simulink model "lvpp2d"  (Simulink 8.4)
settings: Solver=ode45  SolverMode=SingleTasking  StartTime=0.0  StopTime=20  RelTol=1e-3  AbsTol=1e-6
settings Model: Creator=The MathWorks Inc.  LastModifiedBy=gcampa  ExtModeTrigMode=oneshot  ExtModeArmWhenConnect=off
settings DataIOCC: ExternalInput=[]  InitialState=[]  LimitDataPoints=off  SaveOutput=off  SaveTime=off
settings OptimizationCC: BlockReduction=off  BooleanDataType=off  ExpressionDepthLimit=128  InitFltsAndDblsToZero=on
settings DebuggingCC: SaveWithParameterizedLinksMsg=none  SignalResolutionControl=TryResolveAllWithWarning  SolverPrmCheckMsg=none  MultiTaskDSMMsg=warning  MultiTaskCondExecSysMsg=none  IntegerOverflowMsg=none  FcnCallInpInsideContextMsg=EnableAllAsError  FrameProcessingCompatibilityMsg=error  StateNameClashWarn=none
settings HardwareCC: TargetUnknown=on
settings GRTTargetCC: TargetFcnLib=ansi_tfl_tmw.mat
settings ConfigComp: CovMetricSettings=dw  CovHtmlReporting=on  CovSaveCumulativeToWorkspaceVar=on  CovSaveSingleToWorkspaceVar=on  CovModelRefEnable=Off  CovExternalEMLEnable=off  CovSFcnEnable=off

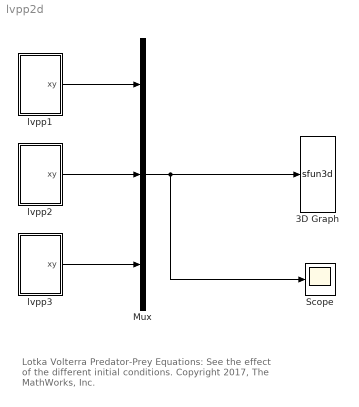
== system lvpp2d ==
  note: Lotka Volterra Predator-Prey Equations:
      | See the effect of the different initial conditions.
      | Copyright 2017, The MathWorks, Inc.
  3D Graph : S-Function  LoadFcn=if exist('sfun3d','file'), sfun3d([],[],[],'LoadBlock'); end  FunctionName=sfun3d  Parameters=ax,T,np,cp,gd,ls,mk,mx,hd,tb  EnableBusSupport=off  mask(3D Graph){np=3, ax=[0 200 0 400 0 1], mx=2000, T=0.01, cp=[0 0 10], gd=on, hd=on, tb=off, ls=-, mk=none}
      mask prompts: np "Number of moving points (lines)"; ax "Range: [xmin xmax  ymin ymax zmin zmax]"; mx "Max number of points in each line"; T "Sampling Time"; cp "Camera position (use [0 0 1] for 2D XY view)"; gd "Grid (on|off)"; hd "HeadMarkers (on|off)"; tb "Toolbar (on|off)"; ls "LineStyle"; mk "LineMarker"
      mask help:
      | This block plots the position of several points in the XYZ space. The input contains the coordinates of all the points (x1,y1,z1,x2,y2,z2,...).
      | The number of moving points (lines), the XYZ ranges, sampling time, camera position, and grid (among other things) can be set as mask parameters.
      settings: CopyFcn=if exist('sfun3d','file'), sfun3d([],[],[],'CopyBlock'); end  DeleteFcn=if exist('sfun3d','file'), sfun3d([],[],[],'DeleteBlock'); end  NameChangeFcn=if exist('sfun3d','file'), sfun3d([],[],[],'NameChange'); end
      mask Help:
      | This block plots the position of several points in the XYZ space. The input contains the coordinates of all the points (x1,y1,z1,x2,y2,z2,...).
      | The number of moving points (lines), the XYZ ranges, sampling time, camera position, and grid (among other things) can be set as mask parameters.
      mask TypeOptions ls: - | -- | : | -. | none
      mask TypeOptions mk: none | . | + | o | * | x | square | diamond | v | ^ | > | < | pentagram | hexagram
      mask Display: plot([.05 .95 .95 .05 .05],[.45 .45 .95 .95 .45], 0.5+cos(0:0.1:2*pi)*0.3,0.7+sin(0:0.1:2*pi)*0.2)
  Mux : Mux  Inputs=[3 3 3]
  Scope : Scope
      settings: TimeRange=20  YMin=0  YMax=400
  lvpp1 : Subsystem  mask(Lotka Volterra System){a=1, b=0.01, c=1, d=0.02, xy0=[20 20]}
      mask prompts: xy0 "Initial point p0 = [x0 y0]"
      mask help:
      | This autonomous system represents the lotka volterra prey predator model:
      |  xdot =  ax - bxy;   ydot = -cy +dxy
      |  where x represents the prey and y represents the predator.
      |  Parameters and initial state can be selected from the mask.
      mask Help:
      | This autonomous system represents the lotka volterra prey predator model.
      |  <p>
      |  The system equations are:
      |  xdot =  ax - bxy
      |  ydot = -cy +dxy
      |  where x represents the prey and y represents the predator.
      |  Parameters and initial state can be selected from the mask.
  lvpp2 : Subsystem  mask(Lotka Volterra System){a=1, b=0.01, c=1, d=0.02, xy0=[30 60]}
      mask prompts: xy0 "Initial point p0 = [x0 y0]"
      mask help:
      | This autonomous system represents the lotka volterra prey predator model:
      |  xdot =  ax - bxy;   ydot = -cy +dxy
      |  where x represents the prey and y represents the predator.
      |  Parameters and initial state can be selected from the mask.
      mask Help:
      | This autonomous system represents the lotka volterra prey predator model.
      |  <p>
      |  The system equations are:
      |  xdot =  ax - bxy
      |  ydot = -cy +dxy
      |  where x represents the prey and y represents the predator.
      |  Parameters and initial state can be selected from the mask.
  lvpp3 : Subsystem  mask(Lotka Volterra System){a=1, b=0.01, c=1, d=0.02, xy0=[50 100]*0.9}
      mask prompts: xy0 "Initial point p0 = [x0 y0]"
      mask help:
      | This autonomous system represents the lotka volterra prey predator model:
      |  xdot =  ax - bxy;   ydot = -cy +dxy
      |  where x represents the prey and y represents the predator.
      |  Parameters and initial state can be selected from the mask.
      mask Help:
      | This autonomous system represents the lotka volterra prey predator model.
      |  <p>
      |  The system equations are:
      |  xdot =  ax - bxy
      |  ydot = -cy +dxy
      |  where x represents the prey and y represents the predator.
      |  Parameters and initial state can be selected from the mask.
  wires:
  Mux/1 -> 3D Graph/1, Scope/1
  lvpp1/1(xy) -> Mux/1
  lvpp2/1(xy) -> Mux/2
  lvpp3/1(xy) -> Mux/3

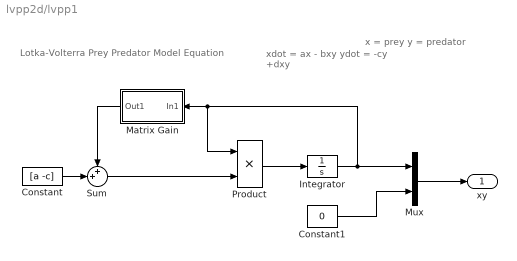
== system lvpp2d/lvpp1 ==
  note: Lotka-Volterra Prey Predator Model Equation
  note: xdot =  ax - bxy
      | ydot = -cy +dxy
  note: x = prey
      | y = predator
  Constant : Constant  Value=[a -c]
  Constant1 : Constant  Value=0
  Integrator : Integrator  InitialCondition=xy0
  Matrix Gain : Subsystem  mask(Matrix Gain){K=[0 -b;d 0]}
      mask prompts: K "Gain matrix:"
      mask help: Matrix Gain.
      mask Help: Multiplies input vector by entered matrix to produce output vector (y=Au).
      mask Display: disp('[0 -b; d 0]')
  Mux : Mux  Inputs=[2 1]
  Product : Product  SaturateOnIntegerOverflow=on  RndMeth=Zero  InputSameDT=on  OutDataTypeStr=Inherit: Same as first input
  Sum : Sum  Inputs=++|  InputSameDT=on  OutDataTypeStr=Inherit: Same as first input
  xy : Outport
  wires:
  Constant/1 -> Sum/2
  Matrix Gain/1(Out1) -> Sum/1
  Product/1 -> Integrator/1
  Integrator/1 -> Mux/1, Product/1, Matrix Gain/1(In1)
  Sum/1 -> Product/2
  Constant1/1 -> Mux/2
  Mux/1 -> xy/1

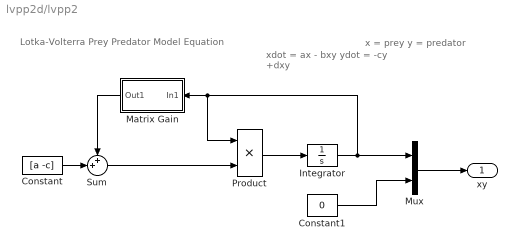
== system lvpp2d/lvpp2 ==
  note: x = prey
      | y = predator
  note: xdot =  ax - bxy
      | ydot = -cy +dxy
  note: Lotka-Volterra Prey Predator Model Equation
  Constant : Constant  Value=[a -c]
  Constant1 : Constant  Value=0
  Integrator : Integrator  InitialCondition=xy0
  Matrix Gain : Subsystem  mask(Matrix Gain){K=[0 -b;d 0]}
      mask prompts: K "Gain matrix:"
      mask help: Matrix Gain.
      mask Help: Multiplies input vector by entered matrix to produce output vector (y=Au).
      mask Display: disp('[0 -b; d 0]')
  Mux : Mux  Inputs=[2 1]
  Product : Product  SaturateOnIntegerOverflow=on  RndMeth=Zero  InputSameDT=on  OutDataTypeStr=Inherit: Same as first input
  Sum : Sum  Inputs=++|  InputSameDT=on  OutDataTypeStr=Inherit: Same as first input
  xy : Outport
  wires:
  Mux/1 -> xy/1
  Constant1/1 -> Mux/2
  Sum/1 -> Product/2
  Integrator/1 -> Matrix Gain/1(In1), Product/1, Mux/1
  Product/1 -> Integrator/1
  Matrix Gain/1(Out1) -> Sum/1
  Constant/1 -> Sum/2

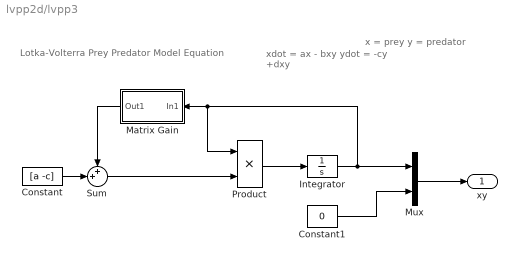
== system lvpp2d/lvpp3 ==
  note: Lotka-Volterra Prey Predator Model Equation
  note: xdot =  ax - bxy
      | ydot = -cy +dxy
  note: x = prey
      | y = predator
  Constant : Constant  Value=[a -c]
  Constant1 : Constant  Value=0
  Integrator : Integrator  InitialCondition=xy0
  Matrix Gain : Subsystem  mask(Matrix Gain){K=[0 -b;d 0]}
      mask prompts: K "Gain matrix:"
      mask help: Matrix Gain.
      mask Help: Multiplies input vector by entered matrix to produce output vector (y=Au).
      mask Display: disp('[0 -b; d 0]')
  Mux : Mux  Inputs=[2 1]
  Product : Product  SaturateOnIntegerOverflow=on  RndMeth=Zero  InputSameDT=on  OutDataTypeStr=Inherit: Same as first input
  Sum : Sum  Inputs=++|  InputSameDT=on  OutDataTypeStr=Inherit: Same as first input
  xy : Outport
  wires:
  Constant/1 -> Sum/2
  Matrix Gain/1(Out1) -> Sum/1
  Product/1 -> Integrator/1
  Integrator/1 -> Mux/1, Product/1, Matrix Gain/1(In1)
  Sum/1 -> Product/2
  Constant1/1 -> Mux/2
  Mux/1 -> xy/1

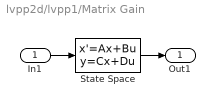
== system lvpp2d/lvpp1/Matrix Gain ==
  In1 : Inport
  State Space : StateSpace  A=[]  B=[]  C=[]  D=K  X0=0
  Out1 : Outport
  wires:
  In1/1 -> State Space/1
  State Space/1 -> Out1/1

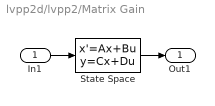
== system lvpp2d/lvpp2/Matrix Gain ==
  In1 : Inport
  State Space : StateSpace  A=[]  B=[]  C=[]  D=K  X0=0
  Out1 : Outport
  wires:
  State Space/1 -> Out1/1
  In1/1 -> State Space/1

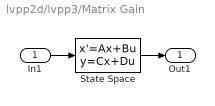
== system lvpp2d/lvpp3/Matrix Gain ==
  In1 : Inport
  State Space : StateSpace  A=[]  B=[]  C=[]  D=K  X0=0
  Out1 : Outport
  wires:
  In1/1 -> State Space/1
  State Space/1 -> Out1/1
